simulink model "model"  (R2024b)
settings: Solver=VariableStepAuto  StartTime=0.0  StopTime=1  RelTol=1e-3
values from neighbouring files (symbols this model uses):
  A = [0 1 0 0; 0 0 a12 0; 0 0 0 1; 0 0 a32 0]    [balancing_robot.m]
  B = [0; b1; 0; b2]    [balancing_robot.m]
  C = [1 0 0 0; 0 0 1 0]    [balancing_robot.m]
  D = [0; 0]    [balancing_robot.m]
libraries: simulink x3, cstblocks x2, slpidlib x1
settings Model: Creator=manuel  LastModifiedBy=manuel

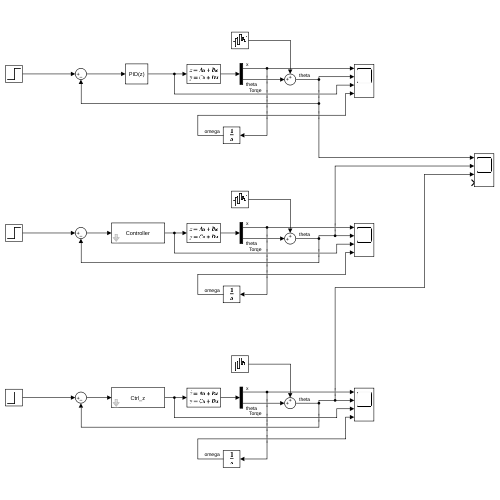
[thumbnail: Simulink's stored preview of the top-level diagram]
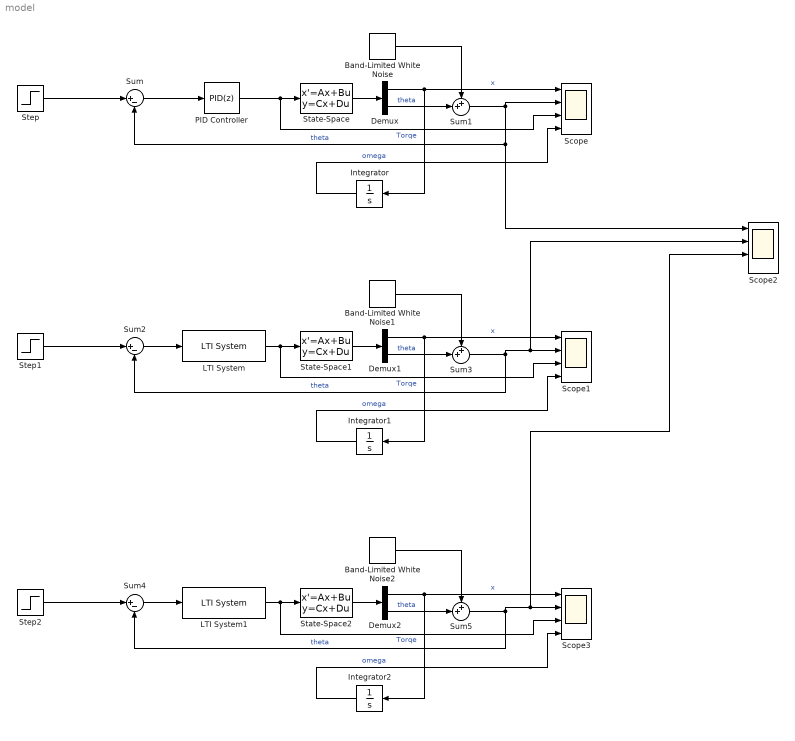
== system model ==
  Band-Limited White Noise : simulink/Sources/Band-Limited White Noise  Cov=[0.0001]  Ts=0.1  seed=[23341]
  Band-Limited White Noise1 : simulink/Sources/Band-Limited White Noise  Cov=[0.0001]  Ts=0.1  seed=[23341]
  Band-Limited White Noise2 : simulink/Sources/Band-Limited White Noise  Cov=[0.0001]  Ts=0.1  seed=[23341]
  Demux : Demux  Outputs=2
  Demux1 : Demux  Outputs=2
  Demux2 : Demux  Outputs=2
  Integrator : Integrator
  Integrator1 : Integrator
  Integrator2 : Integrator
  LTI System : cstblocks/LTI System  sys=Controller  IC=[]  PadeOrder=0
  LTI System1 : cstblocks/LTI System  sys=Ctrl_z  IC=[]  PadeOrder=0
  PID Controller : slpidlib/PID Controller  Controller=PID  Form=Parallel  TimeDomain=Discrete-time  UseExternalTs=off  SampleTime=0.001  IntegratorMethod=Forward Euler  FilterMethod=Forward Euler  ControllerParametersSource=internal  P=1.5  I=0.1  UseKiTs=off  D=0.03  UseExternalDerivativeSource=off  N=100  UseFilter=on  TunerSelectOption=Transfer Function Based (PID Tuner App)  InitialConditionSource=internal  InitialConditionForIntegrator=0  InitialConditionForFilter=0  DifferentiatorICPrevScaledInput=0  ExternalReset=none  TrackingMode=off  Kt=1  LimitOutput=off  SatLimitsSource=internal  UpperSaturationLimit=inf  LowerSaturationLimit=-inf  LinearizeAsGain=on  AntiWindupMode=none  Kb=1  LimitIntegrator=off  UpperIntegratorSaturationLimit=inf  LowerIntegratorSaturationLimit=-inf  POutMin=[]  POutMax=[]  IOutMin=[]  IOutMax=[]  DOutMin=[]  DOutMax=[]  NOutMin=[]  NOutMax=[]  SumOutMin=[]  SumOutMax=[]  SaturationOutMin=[]  SaturationOutMax=[]  PParamMin=[]  PParamMax=[]  IParamMin=[]  IParamMax=[]  DParamMin=[]  DParamMax=[]  NParamMin=[]  NParamMax=[]  KbParamMin=[]  KbParamMax=[]  KtParamMin=[]  KtParamMax=[]  KbOutMin=[]  KbOutMax=[]  KtOutMin=[]  KtOutMax=[]  IntegratorOutMin=[]  IntegratorOutMax=[]  FilterOutMin=[]  FilterOutMax=[]  SumI1OutMin=[]  SumI1OutMax=[]  SumI2OutMin=[]  SumI2OutMax=[]  SumI3OutMin=[]  SumI3OutMax=[]  SumI4OutMin=[]  SumI4OutMax=[]  SumDOutMin=[]  SumDOutMax=[]  DifferentiatorOutMin=[]  DifferentiatorOutMax=[]  FilterDiffOutCoefMin=[]  FilterDiffOutCoefMax=[]  ReciprocalOutMin=[]  ReciprocalOutMax=[]  SumDenOutMin=[]  SumDenOutMax=[]  SumNumOutMin=[]  SumNumOutMax=[]  DivideOutMin=[]  DivideOutMax=[]  UdiffTsProdOutMin=[]  UdiffTsProdOutMax=[]  NTsProdOutMin=[]  NTsProdOutMax=[]  UintegralTsProdOutMin=[]  UintegralTsProdOutMax=[]  UngainTsProdOutMin=[]  UngainTsProdOutMax=[]  ClampingZeroOutDataTypeStr=Inherit: Inherit via back propagation  ClampingZeroOutMin=[]  ClampingZeroOutMax=[]  FilterDenConstantOutDataTypeStr=Inherit: Inherit via back propagation  FilterDenConstantOutMin=[]  FilterDenConstantOutMax=[]  PCopyOutDataTypeStr=Inherit: Inherit via back propagation  PCopyOutMin=[]  PCopyOutMax=[]  NCopyOutDataTypeStr=Inherit: Inherit via back propagation  NCopyOutMin=[]  NCopyOutMax=[]  IntegratorContinuousStateAttributes=''  IntegratorStateMustResolveToSignalObject=off  IntegratorRTWStateStorageClass=Auto  FilterContinuousStateAttributes=''  FilterStateMustResolveToSignalObject=off  FilterRTWStateStorageClass=Auto  ParallelPVariant=InternalParameters  IdealPVariant=Disabled  IVariant=InternalParameters  DVariant=InternalParameters  IntegratorVariant=Discrete  SatVariant=Disabled  AWVariant=Passthrough  PCopyVariant=Disabled  TRVariant=Disabled  FdbkBlocksVariant=Forward  IdealPFdbkVariant=Disabled  SatFdbkVariant=Disabled  DerivativeFilterVariant=ForwardEulerFilter  NVariant=InternalParameters  NCopyVariant=Disabled  FilterICVariant=InternalICsFilter  IntegratorICVariant=InternalICs  ExternalResetVariant=Disabled  TRSumVariant=Passthrough  SumFdbkVariant=Disabled  SumVariant=Sum_PID  TsampFilterVariant=InternalTs  TsampNgainVariant=Passthrough  TsampIntegralVariant=Disabled_SignalSpec  ExternalSaturationOutDataTypeStr=Inherit: Same as second input  DerivativeSourceVariant=ErrorSignal  PreIntVariant=InternalPreInt
  Scope{,1..3} (4 alike) : Scope  NumInputPorts=4
  State-Space : StateSpace  A=A  B=B  C=C  D=D  InitialCondition=[0 0 pi/8 0]
  State-Space1 : StateSpace  A=A  B=B  C=C  D=D  InitialCondition=[0 0 pi/8 0]
  State-Space2 : StateSpace  A=A  B=B  C=C  D=D  InitialCondition=[0 0 pi/8 0]
  Step : Step  Time=5  SampleTime=0
  Step1 : Step  Time=5  SampleTime=0
  Step2 : Step  Time=5  SampleTime=0
  Sum : Sum  Inputs=|+-
  Sum1 : Sum  Inputs=++|
  Sum2 : Sum  Inputs=|+-
  Sum3 : Sum  Inputs=++|
  Sum4 : Sum  Inputs=|+-
  Sum5 : Sum  Inputs=++|
  wires:
  Step/1 -> Sum/1
  Sum/1 -> PID Controller/1
  PID Controller/1 -> Scope/3, State-Space/1  "Torqe"
  State-Space/1 -> Demux/1
  Sum1/1 -> Scope2/1, Sum/2, Scope/2  "theta"
  Demux/1 -> Integrator/1, Scope/1  "x"
  Integrator/1 -> Scope/4  "omega"
  Demux/2 -> Sum1/2  "theta"
  Band-Limited White Noise/1 -> Sum1/1
  LTI System/1 -> Scope1/3, State-Space1/1  "Torqe"
  Sum2/1 -> LTI System/1
  Step1/1 -> Sum2/1
  State-Space1/1 -> Demux1/1
  Band-Limited White Noise1/1 -> Sum3/1
  Demux1/2 -> Sum3/2  "theta"
  Demux1/1 -> Integrator1/1, Scope1/1  "x"
  Sum3/1 -> Sum2/2, Scope2/2, Scope1/2  "theta"
  Integrator1/1 -> Scope1/4  "omega"
  Sum5/1 -> Sum4/2, Scope2/3, Scope3/2  "theta"
  Demux2/1 -> Integrator2/1, Scope3/1  "x"
  State-Space2/1 -> Demux2/1
  Step2/1 -> Sum4/1
  Demux2/2 -> Sum5/2  "theta"
  Band-Limited White Noise2/1 -> Sum5/1
  Integrator2/1 -> Scope3/4  "omega"
  Sum4/1 -> LTI System1/1
  LTI System1/1 -> Scope3/3, State-Space2/1  "Torqe"
